simulink model "VCU_CS75_12_27_test"  (R2014a)
settings: Solver=FixedStepDiscrete  StartTime=0.0  StopTime=25  FixedStep=0.0005  RelTol=1e-3
undefined symbols (not defined in the file): D1, D2, D3, ecucoder_acal, ErrorSumMax1, ErrorSumMax2, ErrorSumMax3, I1, I2, I3, I_SW01_L, LaterlAngleCommand, LDW, P1, P2, P3, RemoteAcclPosition
libraries: simulink x913, ec5744lib x39
(part 26 of 30)

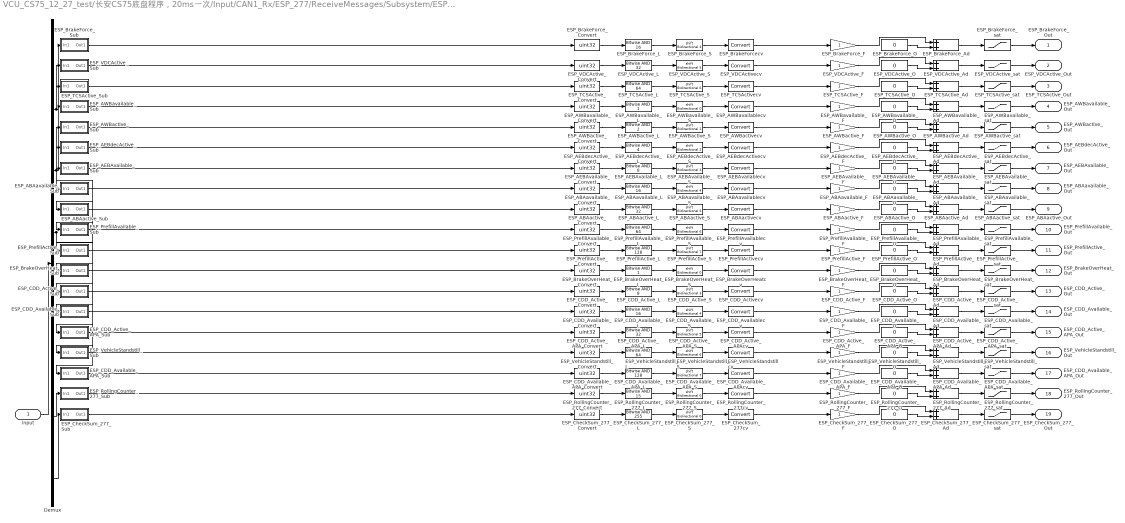
== system VCU_CS75_12_27_test/长安CS75底盘程序，20ms一次/Input/CAN1_Rx/ESP_277/ReceiveMessages/Subsystem/ESP_1 ==
  input : Inport
  Demux : Demux  Outputs=8
  ESP_ABAactive_Ad : Sum
  ESP_ABAactive_Convert : DataTypeConversion  OutDataTypeStr=uint32
  ESP_ABAactive_F : Gain
  ESP_ABAactive_L : simulink/Logic and Bit Operations/Bitwise Operator  logicop=AND  UseBitMask=on  BitMask=32  BitMaskRealWorld=Stored Integer
  ESP_ABAactive_O : Constant  Value=0  OutDataTypeStr=single
  ESP_ABAactive_S : ArithShift  BitShiftNumber=5
  ESP_ABAactive_Sub : Subsystem
  ESP_ABAactive_sat : Saturate  UpperLimit=1  LowerLimit=0
  ESP_ABAactivecv : DataTypeConversion
  ESP_ABAavailable_Ad : Sum
  ESP_ABAavailable_Convert : DataTypeConversion  OutDataTypeStr=uint32
  ESP_ABAavailable_F : Gain
  ESP_ABAavailable_L : simulink/Logic and Bit Operations/Bitwise Operator  logicop=AND  UseBitMask=on  BitMask=16  BitMaskRealWorld=Stored Integer
  ESP_ABAavailable_O : Constant  Value=0  OutDataTypeStr=single
  ESP_ABAavailable_S : ArithShift  BitShiftNumber=4
  ESP_ABAavailable_Sub : Subsystem
  ESP_ABAavailable_sat : Saturate  UpperLimit=1  LowerLimit=0
  ESP_ABAavailablecv : DataTypeConversion
  ESP_AEBAvailable_Ad : Sum
  ESP_AEBAvailable_Convert : DataTypeConversion  OutDataTypeStr=uint32
  ESP_AEBAvailable_F : Gain
  ESP_AEBAvailable_L : simulink/Logic and Bit Operations/Bitwise Operator  logicop=AND  UseBitMask=on  BitMask=8  BitMaskRealWorld=Stored Integer
  ESP_AEBAvailable_O : Constant  Value=0  OutDataTypeStr=single
  ESP_AEBAvailable_S : ArithShift  BitShiftNumber=3
  ESP_AEBAvailable_Sub : Subsystem
  ESP_AEBAvailable_sat : Saturate  UpperLimit=1  LowerLimit=0
  ESP_AEBAvailablecv : DataTypeConversion
  ESP_AEBdecActive_Ad : Sum
  ESP_AEBdecActive_Convert : DataTypeConversion  OutDataTypeStr=uint32
  ESP_AEBdecActive_F : Gain
  ESP_AEBdecActive_L : simulink/Logic and Bit Operations/Bitwise Operator  logicop=AND  UseBitMask=on  BitMask=4  BitMaskRealWorld=Stored Integer
  ESP_AEBdecActive_O : Constant  Value=0  OutDataTypeStr=single
  ESP_AEBdecActive_S : ArithShift  BitShiftNumber=2
  ESP_AEBdecActive_Sub : Subsystem
  ESP_AEBdecActive_sat : Saturate  UpperLimit=1  LowerLimit=0
  ESP_AEBdecActivecv : DataTypeConversion
  ESP_AWBactive_Ad : Sum
  ESP_AWBactive_Convert : DataTypeConversion  OutDataTypeStr=uint32
  ESP_AWBactive_F : Gain
  ESP_AWBactive_L : simulink/Logic and Bit Operations/Bitwise Operator  logicop=AND  UseBitMask=on  BitMask=2  BitMaskRealWorld=Stored Integer
  ESP_AWBactive_O : Constant  Value=0  OutDataTypeStr=single
  ESP_AWBactive_S : ArithShift  BitShiftNumber=1
  ESP_AWBactive_Sub : Subsystem
  ESP_AWBactive_sat : Saturate  UpperLimit=1  LowerLimit=0
  ESP_AWBactivecv : DataTypeConversion
  ESP_AWBavailable_Ad : Sum
  ESP_AWBavailable_Convert : DataTypeConversion  OutDataTypeStr=uint32
  ESP_AWBavailable_F : Gain
  ESP_AWBavailable_L : simulink/Logic and Bit Operations/Bitwise Operator  logicop=AND  UseBitMask=on  BitMask=1  BitMaskRealWorld=Stored Integer
  ESP_AWBavailable_O : Constant  Value=0  OutDataTypeStr=single
  ESP_AWBavailable_S : ArithShift
  ESP_AWBavailable_Sub : Subsystem
  ESP_AWBavailable_sat : Saturate  UpperLimit=1  LowerLimit=0
  ESP_AWBavailablecv : DataTypeConversion
  ESP_BrakeForce_Ad : Sum
  ESP_BrakeForce_Convert : DataTypeConversion  OutDataTypeStr=uint32
  ESP_BrakeForce_F : Gain
  ESP_BrakeForce_L : simulink/Logic and Bit Operations/Bitwise Operator  logicop=AND  UseBitMask=on  BitMask=16  BitMaskRealWorld=Stored Integer
  ESP_BrakeForce_O : Constant  Value=0  OutDataTypeStr=single
  ESP_BrakeForce_S : ArithShift  BitShiftNumber=4
  ESP_BrakeForce_Sub : Subsystem
  ESP_BrakeForce_sat : Saturate  UpperLimit=1  LowerLimit=0
  ESP_BrakeForcecv : DataTypeConversion
  ESP_BrakeOverHeat_Ad : Sum
  ESP_BrakeOverHeat_Convert : DataTypeConversion  OutDataTypeStr=uint32
  ESP_BrakeOverHeat_F : Gain
  ESP_BrakeOverHeat_L : simulink/Logic and Bit Operations/Bitwise Operator  logicop=AND  UseBitMask=on  BitMask=1  BitMaskRealWorld=Stored Integer
  ESP_BrakeOverHeat_O : Constant  Value=0  OutDataTypeStr=single
  ESP_BrakeOverHeat_S : ArithShift
  ESP_BrakeOverHeat_Sub : Subsystem
  ESP_BrakeOverHeat_sat : Saturate  UpperLimit=1  LowerLimit=0
  ESP_BrakeOverHeatcv : DataTypeConversion
  ESP_CDD_Active_APA_Ad : Sum
  ESP_CDD_Active_APA_Convert : DataTypeConversion  OutDataTypeStr=uint32
  ESP_CDD_Active_APA_F : Gain
  ESP_CDD_Active_APA_L : simulink/Logic and Bit Operations/Bitwise Operator  logicop=AND  UseBitMask=on  BitMask=32  BitMaskRealWorld=Stored Integer
  ESP_CDD_Active_APA_O : Constant  Value=0  OutDataTypeStr=single
  ESP_CDD_Active_APA_S : ArithShift  BitShiftNumber=5
  ESP_CDD_Active_APA_Sub : Subsystem
  ESP_CDD_Active_APA_sat : Saturate  UpperLimit=0  LowerLimit=0
  ESP_CDD_Active_APAcv : DataTypeConversion
  ESP_CDD_Active_Ad : Sum
  ESP_CDD_Active_Convert : DataTypeConversion  OutDataTypeStr=uint32
  ESP_CDD_Active_F : Gain
  ESP_CDD_Active_L : simulink/Logic and Bit Operations/Bitwise Operator  logicop=AND  UseBitMask=on  BitMask=8  BitMaskRealWorld=Stored Integer
  ESP_CDD_Active_O : Constant  Value=0  OutDataTypeStr=single
  ESP_CDD_Active_S : ArithShift  BitShiftNumber=3
  ESP_CDD_Active_Sub : Subsystem
  ESP_CDD_Active_sat : Saturate  UpperLimit=1  LowerLimit=0
  ESP_CDD_Activecv : DataTypeConversion
  ESP_CDD_Available_APA_Ad : Sum
  ESP_CDD_Available_APA_Convert : DataTypeConversion  OutDataTypeStr=uint32
  ESP_CDD_Available_APA_F : Gain
  ESP_CDD_Available_APA_L : simulink/Logic and Bit Operations/Bitwise Operator  logicop=AND  UseBitMask=on  BitMask=128  BitMaskRealWorld=Stored Integer
  ESP_CDD_Available_APA_O : Constant  Value=0  OutDataTypeStr=single
  ESP_CDD_Available_APA_S : ArithShift  BitShiftNumber=7
  ESP_CDD_Available_APA_Sub : Subsystem
  ESP_CDD_Available_APA_sat : Saturate  UpperLimit=0  LowerLimit=0
  ESP_CDD_Available_APAcv : DataTypeConversion
  ESP_CDD_Available_Ad : Sum
  ESP_CDD_Available_Convert : DataTypeConversion  OutDataTypeStr=uint32
  ESP_CDD_Available_F : Gain
  ESP_CDD_Available_L : simulink/Logic and Bit Operations/Bitwise Operator  logicop=AND  UseBitMask=on  BitMask=16  BitMaskRealWorld=Stored Integer
  ESP_CDD_Available_O : Constant  Value=0  OutDataTypeStr=single
  ESP_CDD_Available_S : ArithShift  BitShiftNumber=4
  ESP_CDD_Available_Sub : Subsystem
  ESP_CDD_Available_sat : Saturate  UpperLimit=1  LowerLimit=0
  ESP_CDD_Availablecv : DataTypeConversion
  ESP_CheckSum_277_Ad : Sum
  ESP_CheckSum_277_Convert : DataTypeConversion  OutDataTypeStr=uint32
  ESP_CheckSum_277_F : Gain
  ESP_CheckSum_277_L : simulink/Logic and Bit Operations/Bitwise Operator  logicop=AND  UseBitMask=on  BitMask=255  BitMaskRealWorld=Stored Integer
  ESP_CheckSum_277_O : Constant  Value=0  OutDataTypeStr=single
  ESP_CheckSum_277_S : ArithShift
  ESP_CheckSum_277_Sub : Subsystem
  ESP_CheckSum_277_sat : Saturate  UpperLimit=255  LowerLimit=0
  ESP_CheckSum_277cv : DataTypeConversion
  ESP_PrefillActive_Ad : Sum
  ESP_PrefillActive_Convert : DataTypeConversion  OutDataTypeStr=uint32
  ESP_PrefillActive_F : Gain
  ESP_PrefillActive_L : simulink/Logic and Bit Operations/Bitwise Operator  logicop=AND  UseBitMask=on  BitMask=128  BitMaskRealWorld=Stored Integer
  ESP_PrefillActive_O : Constant  Value=0  OutDataTypeStr=single
  ESP_PrefillActive_S : ArithShift  BitShiftNumber=7
  ESP_PrefillActive_Sub : Subsystem
  ESP_PrefillActive_sat : Saturate  UpperLimit=1  LowerLimit=0
  ESP_PrefillActivecv : DataTypeConversion
  ESP_PrefillAvailable_Ad : Sum
  ESP_PrefillAvailable_Convert : DataTypeConversion  OutDataTypeStr=uint32
  ESP_PrefillAvailable_F : Gain
  ESP_PrefillAvailable_L : simulink/Logic and Bit Operations/Bitwise Operator  logicop=AND  UseBitMask=on  BitMask=64  BitMaskRealWorld=Stored Integer
  ESP_PrefillAvailable_O : Constant  Value=0  OutDataTypeStr=single
  ESP_PrefillAvailable_S : ArithShift  BitShiftNumber=6
  ESP_PrefillAvailable_Sub : Subsystem
  ESP_PrefillAvailable_sat : Saturate  UpperLimit=1  LowerLimit=0
  ESP_PrefillAvailablecv : DataTypeConversion
  ESP_RollingCounter_277_Ad : Sum
  ESP_RollingCounter_277_Convert : DataTypeConversion  OutDataTypeStr=uint32
  ESP_RollingCounter_277_F : Gain
  ESP_RollingCounter_277_L : simulink/Logic and Bit Operations/Bitwise Operator  logicop=AND  UseBitMask=on  BitMask=15  BitMaskRealWorld=Stored Integer
  ESP_RollingCounter_277_O : Constant  Value=0  OutDataTypeStr=single
  ESP_RollingCounter_277_S : ArithShift
  ESP_RollingCounter_277_Sub : Subsystem
  ESP_RollingCounter_277_sat : Saturate  UpperLimit=15  LowerLimit=0
  ESP_RollingCounter_277cv : DataTypeConversion
  ESP_TCSActive_Ad : Sum
  ESP_TCSActive_Convert : DataTypeConversion  OutDataTypeStr=uint32
  ESP_TCSActive_F : Gain
  ESP_TCSActive_L : simulink/Logic and Bit Operations/Bitwise Operator  logicop=AND  UseBitMask=on  BitMask=64  BitMaskRealWorld=Stored Integer
  ESP_TCSActive_O : Constant  Value=0  OutDataTypeStr=single
  ESP_TCSActive_S : ArithShift  BitShiftNumber=6
  ESP_TCSActive_Sub : Subsystem
  ESP_TCSActive_sat : Saturate  UpperLimit=1  LowerLimit=0
  ESP_TCSActivecv : DataTypeConversion
  ESP_VDCActive_Ad : Sum
  ESP_VDCActive_Convert : DataTypeConversion  OutDataTypeStr=uint32
  ESP_VDCActive_F : Gain
  ESP_VDCActive_L : simulink/Logic and Bit Operations/Bitwise Operator  logicop=AND  UseBitMask=on  BitMask=32  BitMaskRealWorld=Stored Integer
  ESP_VDCActive_O : Constant  Value=0  OutDataTypeStr=single
  ESP_VDCActive_S : ArithShift  BitShiftNumber=5
  ESP_VDCActive_Sub : Subsystem
  ESP_VDCActive_sat : Saturate  UpperLimit=1  LowerLimit=0
  ESP_VDCActivecv : DataTypeConversion
  ESP_VehicleStandstill_Ad : Sum
  ESP_VehicleStandstill_Convert : DataTypeConversion  OutDataTypeStr=uint32
  ESP_VehicleStandstill_F : Gain
  ESP_VehicleStandstill_L : simulink/Logic and Bit Operations/Bitwise Operator  logicop=AND  UseBitMask=on  BitMask=64  BitMaskRealWorld=Stored Integer
  ESP_VehicleStandstill_O : Constant  Value=0  OutDataTypeStr=single
  ESP_VehicleStandstill_S : ArithShift  BitShiftNumber=6
  ESP_VehicleStandstill_Sub : Subsystem
  ESP_VehicleStandstill_sat : Saturate  UpperLimit=1  LowerLimit=0
  ESP_VehicleStandstillcv : DataTypeConversion
  ESP_BrakeForce_Out : Outport
  ESP_VDCActive_Out : Outport  Port=2
  ESP_TCSActive_Out : Outport  Port=3
  ESP_AWBavailable_Out : Outport  Port=4
  ESP_AWBactive_Out : Outport  Port=5
  ESP_AEBdecActive_Out : Outport  Port=6
  ESP_AEBAvailable_Out : Outport  Port=7
  ESP_ABAavailable_Out : Outport  Port=8
  ESP_ABAactive_Out : Outport  Port=9
  ESP_PrefillAvailable_Out : Outport  Port=10
  ESP_PrefillActive_Out : Outport  Port=11
  ESP_BrakeOverHeat_Out : Outport  Port=12
  ESP_CDD_Active_Out : Outport  Port=13
  ESP_CDD_Available_Out : Outport  Port=14
  ESP_CDD_Active_APA_Out : Outport  Port=15
  ESP_VehicleStandstill_Out : Outport  Port=16
  ESP_CDD_Available_APA_Out : Outport  Port=17
  ESP_RollingCounter_277_Out : Outport  Port=18
  ESP_CheckSum_277_Out : Outport  Port=19
  wires:
  input/1 -> Demux/1
  ESP_CheckSum_277cv/1 -> ESP_CheckSum_277_F/1
  ESP_CheckSum_277_S/1 -> ESP_CheckSum_277cv/1
  ESP_CheckSum_277_L/1 -> ESP_CheckSum_277_S/1
  ESP_CheckSum_277_Convert/1 -> ESP_CheckSum_277_L/1
  ESP_CheckSum_277_Sub/1(Out1) -> ESP_CheckSum_277_Convert/1
  Demux/8 -> ESP_CheckSum_277_Sub/1(In1)
  ESP_CheckSum_277_sat/1 -> ESP_CheckSum_277_Out/1
  ESP_CheckSum_277_Ad/1 -> ESP_CheckSum_277_sat/1
  ESP_CheckSum_277_O/1 -> ESP_CheckSum_277_Ad/2
  ESP_CheckSum_277_F/1 -> ESP_CheckSum_277_Ad/1
  ESP_RollingCounter_277cv/1 -> ESP_RollingCounter_277_F/1
  ESP_RollingCounter_277_S/1 -> ESP_RollingCounter_277cv/1
  ESP_RollingCounter_277_L/1 -> ESP_RollingCounter_277_S/1
  ESP_RollingCounter_277_Convert/1 -> ESP_RollingCounter_277_L/1
  ESP_RollingCounter_277_Sub/1(Out1) -> ESP_RollingCounter_277_Convert/1
  Demux/7 -> ESP_RollingCounter_277_Sub/1(In1)
  ESP_RollingCounter_277_sat/1 -> ESP_RollingCounter_277_Out/1
  ESP_RollingCounter_277_Ad/1 -> ESP_RollingCounter_277_sat/1
  ESP_RollingCounter_277_O/1 -> ESP_RollingCounter_277_Ad/2
  ESP_RollingCounter_277_F/1 -> ESP_RollingCounter_277_Ad/1
  ESP_CDD_Available_APAcv/1 -> ESP_CDD_Available_APA_F/1
  ESP_CDD_Available_APA_S/1 -> ESP_CDD_Available_APAcv/1
  ESP_CDD_Available_APA_L/1 -> ESP_CDD_Available_APA_S/1
  ESP_CDD_Available_APA_Convert/1 -> ESP_CDD_Available_APA_L/1
  ESP_CDD_Available_APA_Sub/1(Out1) -> ESP_CDD_Available_APA_Convert/1
  ESP_CDD_Available_APA_sat/1 -> ESP_CDD_Available_APA_Out/1
  ESP_CDD_Available_APA_Ad/1 -> ESP_CDD_Available_APA_sat/1
  ESP_CDD_Available_APA_O/1 -> ESP_CDD_Available_APA_Ad/2
  ESP_CDD_Available_APA_F/1 -> ESP_CDD_Available_APA_Ad/1
  ESP_VehicleStandstillcv/1 -> ESP_VehicleStandstill_F/1
  ESP_VehicleStandstill_S/1 -> ESP_VehicleStandstillcv/1
  ESP_VehicleStandstill_L/1 -> ESP_VehicleStandstill_S/1
  ESP_VehicleStandstill_Convert/1 -> ESP_VehicleStandstill_L/1
  ESP_VehicleStandstill_Sub/1(Out1) -> ESP_VehicleStandstill_Convert/1
  ESP_VehicleStandstill_sat/1 -> ESP_VehicleStandstill_Out/1
  ESP_VehicleStandstill_Ad/1 -> ESP_VehicleStandstill_sat/1
  ESP_VehicleStandstill_O/1 -> ESP_VehicleStandstill_Ad/2
  ESP_VehicleStandstill_F/1 -> ESP_VehicleStandstill_Ad/1
  ESP_CDD_Active_APAcv/1 -> ESP_CDD_Active_APA_F/1
  ESP_CDD_Active_APA_S/1 -> ESP_CDD_Active_APAcv/1
  ESP_CDD_Active_APA_L/1 -> ESP_CDD_Active_APA_S/1
  ESP_CDD_Active_APA_Convert/1 -> ESP_CDD_Active_APA_L/1
  ESP_CDD_Active_APA_Sub/1(Out1) -> ESP_CDD_Active_APA_Convert/1
  ESP_CDD_Active_APA_sat/1 -> ESP_CDD_Active_APA_Out/1
  ESP_CDD_Active_APA_Ad/1 -> ESP_CDD_Active_APA_sat/1
  ESP_CDD_Active_APA_O/1 -> ESP_CDD_Active_APA_Ad/2
  ESP_CDD_Active_APA_F/1 -> ESP_CDD_Active_APA_Ad/1
  ESP_CDD_Availablecv/1 -> ESP_CDD_Available_F/1
  ESP_CDD_Available_S/1 -> ESP_CDD_Availablecv/1
  ESP_CDD_Available_L/1 -> ESP_CDD_Available_S/1
  ESP_CDD_Available_Convert/1 -> ESP_CDD_Available_L/1
  ESP_CDD_Available_Sub/1(Out1) -> ESP_CDD_Available_Convert/1
  ESP_CDD_Available_sat/1 -> ESP_CDD_Available_Out/1
  ESP_CDD_Available_Ad/1 -> ESP_CDD_Available_sat/1
  ESP_CDD_Available_O/1 -> ESP_CDD_Available_Ad/2
  ESP_CDD_Available_F/1 -> ESP_CDD_Available_Ad/1
  ESP_CDD_Activecv/1 -> ESP_CDD_Active_F/1
  ESP_CDD_Active_S/1 -> ESP_CDD_Activecv/1
  ESP_CDD_Active_L/1 -> ESP_CDD_Active_S/1
  ESP_CDD_Active_Convert/1 -> ESP_CDD_Active_L/1
  ESP_CDD_Active_Sub/1(Out1) -> ESP_CDD_Active_Convert/1
  ESP_CDD_Active_sat/1 -> ESP_CDD_Active_Out/1
  ESP_CDD_Active_Ad/1 -> ESP_CDD_Active_sat/1
  ESP_CDD_Active_O/1 -> ESP_CDD_Active_Ad/2
  ESP_CDD_Active_F/1 -> ESP_CDD_Active_Ad/1
  ESP_BrakeOverHeatcv/1 -> ESP_BrakeOverHeat_F/1
  ESP_BrakeOverHeat_S/1 -> ESP_BrakeOverHeatcv/1
  ESP_BrakeOverHeat_L/1 -> ESP_BrakeOverHeat_S/1
  ESP_BrakeOverHeat_Convert/1 -> ESP_BrakeOverHeat_L/1
  ESP_BrakeOverHeat_Sub/1(Out1) -> ESP_BrakeOverHeat_Convert/1
  Demux/4 -> ESP_CDD_Available_APA_Sub/1(In1), ESP_VehicleStandstill_Sub/1(In1), ESP_CDD_Active_APA_Sub/1(In1), ESP_CDD_Available_Sub/1(In1), ESP_CDD_Active_Sub/1(In1), ESP_BrakeOverHeat_Sub/1(In1)
  ESP_BrakeOverHeat_sat/1 -> ESP_BrakeOverHeat_Out/1
  ESP_BrakeOverHeat_Ad/1 -> ESP_BrakeOverHeat_sat/1
  ESP_BrakeOverHeat_O/1 -> ESP_BrakeOverHeat_Ad/2
  ESP_BrakeOverHeat_F/1 -> ESP_BrakeOverHeat_Ad/1
  ESP_PrefillActivecv/1 -> ESP_PrefillActive_F/1
  ESP_PrefillActive_S/1 -> ESP_PrefillActivecv/1
  ESP_PrefillActive_L/1 -> ESP_PrefillActive_S/1
  ESP_PrefillActive_Convert/1 -> ESP_PrefillActive_L/1
  ESP_PrefillActive_Sub/1(Out1) -> ESP_PrefillActive_Convert/1
  ESP_PrefillActive_sat/1 -> ESP_PrefillActive_Out/1
  ESP_PrefillActive_Ad/1 -> ESP_PrefillActive_sat/1
  ESP_PrefillActive_O/1 -> ESP_PrefillActive_Ad/2
  ESP_PrefillActive_F/1 -> ESP_PrefillActive_Ad/1
  ESP_PrefillAvailablecv/1 -> ESP_PrefillAvailable_F/1
  ESP_PrefillAvailable_S/1 -> ESP_PrefillAvailablecv/1
  ESP_PrefillAvailable_L/1 -> ESP_PrefillAvailable_S/1
  ESP_PrefillAvailable_Convert/1 -> ESP_PrefillAvailable_L/1
  ESP_PrefillAvailable_Sub/1(Out1) -> ESP_PrefillAvailable_Convert/1
  ESP_PrefillAvailable_sat/1 -> ESP_PrefillAvailable_Out/1
  ESP_PrefillAvailable_Ad/1 -> ESP_PrefillAvailable_sat/1
  ESP_PrefillAvailable_O/1 -> ESP_PrefillAvailable_Ad/2
  ESP_PrefillAvailable_F/1 -> ESP_PrefillAvailable_Ad/1
  ESP_ABAactivecv/1 -> ESP_ABAactive_F/1
  ESP_ABAactive_S/1 -> ESP_ABAactivecv/1
  ESP_ABAactive_L/1 -> ESP_ABAactive_S/1
  ESP_ABAactive_Convert/1 -> ESP_ABAactive_L/1
  ESP_ABAactive_Sub/1(Out1) -> ESP_ABAactive_Convert/1
  ESP_ABAactive_sat/1 -> ESP_ABAactive_Out/1
  ESP_ABAactive_Ad/1 -> ESP_ABAactive_sat/1
  ESP_ABAactive_O/1 -> ESP_ABAactive_Ad/2
  ESP_ABAactive_F/1 -> ESP_ABAactive_Ad/1
  ESP_ABAavailablecv/1 -> ESP_ABAavailable_F/1
  ESP_ABAavailable_S/1 -> ESP_ABAavailablecv/1
  ESP_ABAavailable_L/1 -> ESP_ABAavailable_S/1
  ESP_ABAavailable_Convert/1 -> ESP_ABAavailable_L/1
  ESP_ABAavailable_Sub/1(Out1) -> ESP_ABAavailable_Convert/1
  ESP_ABAavailable_sat/1 -> ESP_ABAavailable_Out/1
  ESP_ABAavailable_Ad/1 -> ESP_ABAavailable_sat/1
  ESP_ABAavailable_O/1 -> ESP_ABAavailable_Ad/2
  ESP_ABAavailable_F/1 -> ESP_ABAavailable_Ad/1
  ESP_AEBAvailablecv/1 -> ESP_AEBAvailable_F/1
  ESP_AEBAvailable_S/1 -> ESP_AEBAvailablecv/1
  ESP_AEBAvailable_L/1 -> ESP_AEBAvailable_S/1
  ESP_AEBAvailable_Convert/1 -> ESP_AEBAvailable_L/1
  ESP_AEBAvailable_Sub/1(Out1) -> ESP_AEBAvailable_Convert/1
  ESP_AEBAvailable_sat/1 -> ESP_AEBAvailable_Out/1
  ESP_AEBAvailable_Ad/1 -> ESP_AEBAvailable_sat/1
  ESP_AEBAvailable_O/1 -> ESP_AEBAvailable_Ad/2
  ESP_AEBAvailable_F/1 -> ESP_AEBAvailable_Ad/1
  ESP_AEBdecActivecv/1 -> ESP_AEBdecActive_F/1
  ESP_AEBdecActive_S/1 -> ESP_AEBdecActivecv/1
  ESP_AEBdecActive_L/1 -> ESP_AEBdecActive_S/1
  ESP_AEBdecActive_Convert/1 -> ESP_AEBdecActive_L/1
  ESP_AEBdecActive_Sub/1(Out1) -> ESP_AEBdecActive_Convert/1
  ESP_AEBdecActive_sat/1 -> ESP_AEBdecActive_Out/1
  ESP_AEBdecActive_Ad/1 -> ESP_AEBdecActive_sat/1
  ESP_AEBdecActive_O/1 -> ESP_AEBdecActive_Ad/2
  ESP_AEBdecActive_F/1 -> ESP_AEBdecActive_Ad/1
  ESP_AWBactivecv/1 -> ESP_AWBactive_F/1
  ESP_AWBactive_S/1 -> ESP_AWBactivecv/1
  ESP_AWBactive_L/1 -> ESP_AWBactive_S/1
  ESP_AWBactive_Convert/1 -> ESP_AWBactive_L/1
  ESP_AWBactive_Sub/1(Out1) -> ESP_AWBactive_Convert/1
  ESP_AWBactive_sat/1 -> ESP_AWBactive_Out/1
  ESP_AWBactive_Ad/1 -> ESP_AWBactive_sat/1
  ESP_AWBactive_O/1 -> ESP_AWBactive_Ad/2
  ESP_AWBactive_F/1 -> ESP_AWBactive_Ad/1
  ESP_AWBavailablecv/1 -> ESP_AWBavailable_F/1
  ESP_AWBavailable_S/1 -> ESP_AWBavailablecv/1
  ESP_AWBavailable_L/1 -> ESP_AWBavailable_S/1
  ESP_AWBavailable_Convert/1 -> ESP_AWBavailable_L/1
  ESP_AWBavailable_Sub/1(Out1) -> ESP_AWBavailable_Convert/1
  Demux/3 -> ESP_PrefillActive_Sub/1(In1), ESP_PrefillAvailable_Sub/1(In1), ESP_ABAactive_Sub/1(In1), ESP_ABAavailable_Sub/1(In1), ESP_AEBAvailable_Sub/1(In1), ESP_AEBdecActive_Sub/1(In1), ESP_AWBactive_Sub/1(In1), ESP_AWBavailable_Sub/1(In1)
  ESP_AWBavailable_sat/1 -> ESP_AWBavailable_Out/1
  ESP_AWBavailable_Ad/1 -> ESP_AWBavailable_sat/1
  ESP_AWBavailable_O/1 -> ESP_AWBavailable_Ad/2
  ESP_AWBavailable_F/1 -> ESP_AWBavailable_Ad/1
  ESP_TCSActivecv/1 -> ESP_TCSActive_F/1
  ESP_TCSActive_S/1 -> ESP_TCSActivecv/1
  ESP_TCSActive_L/1 -> ESP_TCSActive_S/1
  ESP_TCSActive_Convert/1 -> ESP_TCSActive_L/1
  ESP_TCSActive_Sub/1(Out1) -> ESP_TCSActive_Convert/1
  ESP_TCSActive_sat/1 -> ESP_TCSActive_Out/1
  ESP_TCSActive_Ad/1 -> ESP_TCSActive_sat/1
  ESP_TCSActive_O/1 -> ESP_TCSActive_Ad/2
  ESP_TCSActive_F/1 -> ESP_TCSActive_Ad/1
  ESP_VDCActivecv/1 -> ESP_VDCActive_F/1
  ESP_VDCActive_S/1 -> ESP_VDCActivecv/1
  ESP_VDCActive_L/1 -> ESP_VDCActive_S/1
  ESP_VDCActive_Convert/1 -> ESP_VDCActive_L/1
  ESP_VDCActive_Sub/1(Out1) -> ESP_VDCActive_Convert/1
  ESP_VDCActive_sat/1 -> ESP_VDCActive_Out/1
  ESP_VDCActive_Ad/1 -> ESP_VDCActive_sat/1
  ESP_VDCActive_O/1 -> ESP_VDCActive_Ad/2
  ESP_VDCActive_F/1 -> ESP_VDCActive_Ad/1
  ESP_BrakeForcecv/1 -> ESP_BrakeForce_F/1
  ESP_BrakeForce_S/1 -> ESP_BrakeForcecv/1
  ESP_BrakeForce_L/1 -> ESP_BrakeForce_S/1
  ESP_BrakeForce_Convert/1 -> ESP_BrakeForce_L/1
  ESP_BrakeForce_Sub/1(Out1) -> ESP_BrakeForce_Convert/1
  Demux/2 -> ESP_TCSActive_Sub/1(In1), ESP_VDCActive_Sub/1(In1), ESP_BrakeForce_Sub/1(In1)
  ESP_BrakeForce_sat/1 -> ESP_BrakeForce_Out/1
  ESP_BrakeForce_Ad/1 -> ESP_BrakeForce_sat/1
  ESP_BrakeForce_O/1 -> ESP_BrakeForce_Ad/2
  ESP_BrakeForce_F/1 -> ESP_BrakeForce_Ad/1

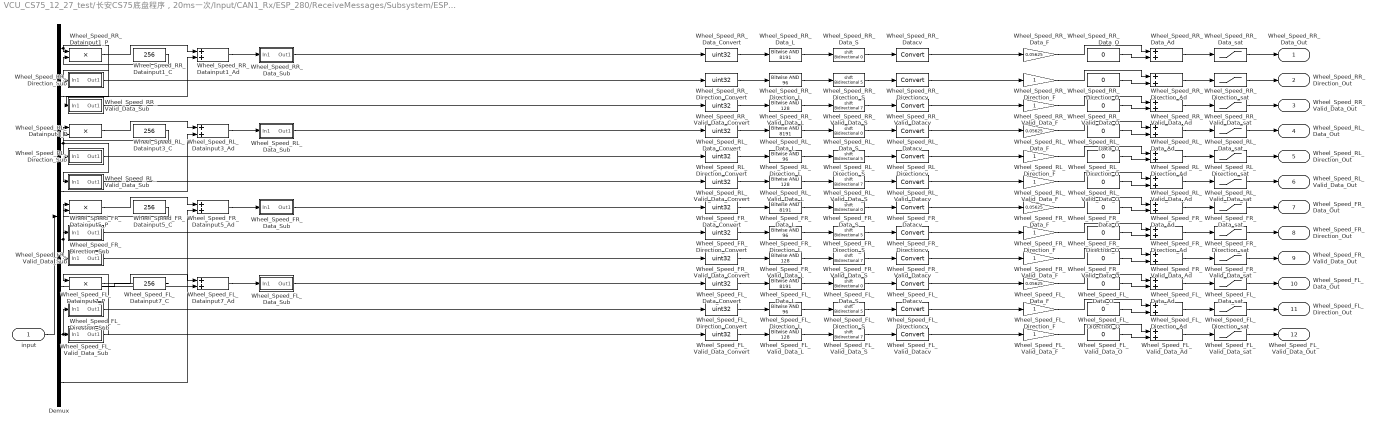
== system VCU_CS75_12_27_test/长安CS75底盘程序，20ms一次/Input/CAN1_Rx/ESP_280/ReceiveMessages/Subsystem/ESP_1 ==
  input : Inport
  Demux : Demux  Outputs=8
  Wheel_Speed_FL_Data_Ad : Sum
  Wheel_Speed_FL_Data_Convert : DataTypeConversion  OutDataTypeStr=uint32
  Wheel_Speed_FL_Data_F : Gain  Gain=0.05625
  Wheel_Speed_FL_Data_L : simulink/Logic and Bit Operations/Bitwise Operator  logicop=AND  UseBitMask=on  BitMask=8191  BitMaskRealWorld=Stored Integer
  Wheel_Speed_FL_Data_O : Constant  Value=0  OutDataTypeStr=single
  Wheel_Speed_FL_Data_S : ArithShift
  Wheel_Speed_FL_Data_Sub : Subsystem
  Wheel_Speed_FL_Data_sat : Saturate  UpperLimit=360  LowerLimit=0
  Wheel_Speed_FL_Datacv : DataTypeConversion
  Wheel_Speed_FL_Datainput7_Ad : Sum
  Wheel_Speed_FL_Datainput7_C : Constant  Value=256
  Wheel_Speed_FL_Datainput7_P : Product
  Wheel_Speed_FL_Direction_Ad : Sum
  Wheel_Speed_FL_Direction_Convert : DataTypeConversion  OutDataTypeStr=uint32
  Wheel_Speed_FL_Direction_F : Gain
  Wheel_Speed_FL_Direction_L : simulink/Logic and Bit Operations/Bitwise Operator  logicop=AND  UseBitMask=on  BitMask=96  BitMaskRealWorld=Stored Integer
  Wheel_Speed_FL_Direction_O : Constant  Value=0  OutDataTypeStr=single
  Wheel_Speed_FL_Direction_S : ArithShift  BitShiftNumber=5
  Wheel_Speed_FL_Direction_Sub : Subsystem
  Wheel_Speed_FL_Direction_sat : Saturate  UpperLimit=3  LowerLimit=0
  Wheel_Speed_FL_Directioncv : DataTypeConversion
  Wheel_Speed_FL_Valid_Data_Ad : Sum
  Wheel_Speed_FL_Valid_Data_Convert : DataTypeConversion  OutDataTypeStr=uint32
  Wheel_Speed_FL_Valid_Data_F : Gain
  Wheel_Speed_FL_Valid_Data_L : simulink/Logic and Bit Operations/Bitwise Operator  logicop=AND  UseBitMask=on  BitMask=128  BitMaskRealWorld=Stored Integer
  Wheel_Speed_FL_Valid_Data_O : Constant  Value=0  OutDataTypeStr=single
  Wheel_Speed_FL_Valid_Data_S : ArithShift  BitShiftNumber=7
  Wheel_Speed_FL_Valid_Data_Sub : Subsystem
  Wheel_Speed_FL_Valid_Data_sat : Saturate  UpperLimit=1  LowerLimit=0
  Wheel_Speed_FL_Valid_Datacv : DataTypeConversion
  Wheel_Speed_FR_Data_Ad : Sum
  Wheel_Speed_FR_Data_Convert : DataTypeConversion  OutDataTypeStr=uint32
  Wheel_Speed_FR_Data_F : Gain  Gain=0.05625
  Wheel_Speed_FR_Data_L : simulink/Logic and Bit Operations/Bitwise Operator  logicop=AND  UseBitMask=on  BitMask=8191  BitMaskRealWorld=Stored Integer
  Wheel_Speed_FR_Data_O : Constant  Value=0  OutDataTypeStr=single
  Wheel_Speed_FR_Data_S : ArithShift
  Wheel_Speed_FR_Data_Sub : Subsystem
  Wheel_Speed_FR_Data_sat : Saturate  UpperLimit=360  LowerLimit=0
  Wheel_Speed_FR_Datacv : DataTypeConversion
  Wheel_Speed_FR_Datainput5_Ad : Sum
  Wheel_Speed_FR_Datainput5_C : Constant  Value=256
  Wheel_Speed_FR_Datainput5_P : Product
  Wheel_Speed_FR_Direction_Ad : Sum
  Wheel_Speed_FR_Direction_Convert : DataTypeConversion  OutDataTypeStr=uint32
  Wheel_Speed_FR_Direction_F : Gain
  Wheel_Speed_FR_Direction_L : simulink/Logic and Bit Operations/Bitwise Operator  logicop=AND  UseBitMask=on  BitMask=96  BitMaskRealWorld=Stored Integer
  Wheel_Speed_FR_Direction_O : Constant  Value=0  OutDataTypeStr=single
  Wheel_Speed_FR_Direction_S : ArithShift  BitShiftNumber=5
  Wheel_Speed_FR_Direction_Sub : Subsystem
  Wheel_Speed_FR_Direction_sat : Saturate  UpperLimit=3  LowerLimit=0
  Wheel_Speed_FR_Directioncv : DataTypeConversion
  Wheel_Speed_FR_Valid_Data_Ad : Sum
  Wheel_Speed_FR_Valid_Data_Convert : DataTypeConversion  OutDataTypeStr=uint32
  Wheel_Speed_FR_Valid_Data_F : Gain
  Wheel_Speed_FR_Valid_Data_L : simulink/Logic and Bit Operations/Bitwise Operator  logicop=AND  UseBitMask=on  BitMask=128  BitMaskRealWorld=Stored Integer
  Wheel_Speed_FR_Valid_Data_O : Constant  Value=0  OutDataTypeStr=single
  Wheel_Speed_FR_Valid_Data_S : ArithShift  BitShiftNumber=7
  Wheel_Speed_FR_Valid_Data_Sub : Subsystem
  Wheel_Speed_FR_Valid_Data_sat : Saturate  UpperLimit=1  LowerLimit=0
  Wheel_Speed_FR_Valid_Datacv : DataTypeConversion
  Wheel_Speed_RL_Data_Ad : Sum
  Wheel_Speed_RL_Data_Convert : DataTypeConversion  OutDataTypeStr=uint32
  Wheel_Speed_RL_Data_F : Gain  Gain=0.05625
  Wheel_Speed_RL_Data_L : simulink/Logic and Bit Operations/Bitwise Operator  logicop=AND  UseBitMask=on  BitMask=8191  BitMaskRealWorld=Stored Integer
  Wheel_Speed_RL_Data_O : Constant  Value=0  OutDataTypeStr=single
  Wheel_Speed_RL_Data_S : ArithShift
  Wheel_Speed_RL_Data_Sub : Subsystem
  Wheel_Speed_RL_Data_sat : Saturate  UpperLimit=360  LowerLimit=0
  Wheel_Speed_RL_Datacv : DataTypeConversion
  Wheel_Speed_RL_Datainput3_Ad : Sum
  Wheel_Speed_RL_Datainput3_C : Constant  Value=256
  Wheel_Speed_RL_Datainput3_P : Product
  Wheel_Speed_RL_Direction_Ad : Sum
  Wheel_Speed_RL_Direction_Convert : DataTypeConversion  OutDataTypeStr=uint32
  Wheel_Speed_RL_Direction_F : Gain
  Wheel_Speed_RL_Direction_L : simulink/Logic and Bit Operations/Bitwise Operator  logicop=AND  UseBitMask=on  BitMask=96  BitMaskRealWorld=Stored Integer
  Wheel_Speed_RL_Direction_O : Constant  Value=0  OutDataTypeStr=single
  Wheel_Speed_RL_Direction_S : ArithShift  BitShiftNumber=5
  Wheel_Speed_RL_Direction_Sub : Subsystem
  Wheel_Speed_RL_Direction_sat : Saturate  UpperLimit=3  LowerLimit=0
  Wheel_Speed_RL_Directioncv : DataTypeConversion
  Wheel_Speed_RL_Valid_Data_Ad : Sum
  Wheel_Speed_RL_Valid_Data_Convert : DataTypeConversion  OutDataTypeStr=uint32
  Wheel_Speed_RL_Valid_Data_F : Gain
  Wheel_Speed_RL_Valid_Data_L : simulink/Logic and Bit Operations/Bitwise Operator  logicop=AND  UseBitMask=on  BitMask=128  BitMaskRealWorld=Stored Integer
  Wheel_Speed_RL_Valid_Data_O : Constant  Value=0  OutDataTypeStr=single
  Wheel_Speed_RL_Valid_Data_S : ArithShift  BitShiftNumber=7
  Wheel_Speed_RL_Valid_Data_Sub : Subsystem
  Wheel_Speed_RL_Valid_Data_sat : Saturate  UpperLimit=1  LowerLimit=0
  Wheel_Speed_RL_Valid_Datacv : DataTypeConversion
  Wheel_Speed_RR_Data_Ad : Sum
  Wheel_Speed_RR_Data_Convert : DataTypeConversion  OutDataTypeStr=uint32
  Wheel_Speed_RR_Data_F : Gain  Gain=0.05625
  Wheel_Speed_RR_Data_L : simulink/Logic and Bit Operations/Bitwise Operator  logicop=AND  UseBitMask=on  BitMask=8191  BitMaskRealWorld=Stored Integer
  Wheel_Speed_RR_Data_O : Constant  Value=0  OutDataTypeStr=single
  Wheel_Speed_RR_Data_S : ArithShift
  Wheel_Speed_RR_Data_Sub : Subsystem
  Wheel_Speed_RR_Data_sat : Saturate  UpperLimit=360  LowerLimit=0
  Wheel_Speed_RR_Datacv : DataTypeConversion
  Wheel_Speed_RR_Datainput1_Ad : Sum
  Wheel_Speed_RR_Datainput1_C : Constant  Value=256
  Wheel_Speed_RR_Datainput1_P : Product
  Wheel_Speed_RR_Direction_Ad : Sum
  Wheel_Speed_RR_Direction_Convert : DataTypeConversion  OutDataTypeStr=uint32
  Wheel_Speed_RR_Direction_F : Gain
  Wheel_Speed_RR_Direction_L : simulink/Logic and Bit Operations/Bitwise Operator  logicop=AND  UseBitMask=on  BitMask=96  BitMaskRealWorld=Stored Integer
  Wheel_Speed_RR_Direction_O : Constant  Value=0  OutDataTypeStr=single
  Wheel_Speed_RR_Direction_S : ArithShift  BitShiftNumber=5
  Wheel_Speed_RR_Direction_Sub : Subsystem
  Wheel_Speed_RR_Direction_sat : Saturate  UpperLimit=3  LowerLimit=0
  Wheel_Speed_RR_Directioncv : DataTypeConversion
  Wheel_Speed_RR_Valid_Data_Ad : Sum
  Wheel_Speed_RR_Valid_Data_Convert : DataTypeConversion  OutDataTypeStr=uint32
  Wheel_Speed_RR_Valid_Data_F : Gain
  Wheel_Speed_RR_Valid_Data_L : simulink/Logic and Bit Operations/Bitwise Operator  logicop=AND  UseBitMask=on  BitMask=128  BitMaskRealWorld=Stored Integer
  Wheel_Speed_RR_Valid_Data_O : Constant  Value=0  OutDataTypeStr=single
  Wheel_Speed_RR_Valid_Data_S : ArithShift  BitShiftNumber=7
  Wheel_Speed_RR_Valid_Data_Sub : Subsystem
  Wheel_Speed_RR_Valid_Data_sat : Saturate  UpperLimit=1  LowerLimit=0
  Wheel_Speed_RR_Valid_Datacv : DataTypeConversion
  Wheel_Speed_RR_Data_Out : Outport
  Wheel_Speed_RR_Direction_Out : Outport  Port=2
  Wheel_Speed_RR_Valid_Data_Out : Outport  Port=3
  Wheel_Speed_RL_Data_Out : Outport  Port=4
  Wheel_Speed_RL_Direction_Out : Outport  Port=5
  Wheel_Speed_RL_Valid_Data_Out : Outport  Port=6
  Wheel_Speed_FR_Data_Out : Outport  Port=7
  Wheel_Speed_FR_Direction_Out : Outport  Port=8
  Wheel_Speed_FR_Valid_Data_Out : Outport  Port=9
  Wheel_Speed_FL_Data_Out : Outport  Port=10
  Wheel_Speed_FL_Direction_Out : Outport  Port=11
  Wheel_Speed_FL_Valid_Data_Out : Outport  Port=12
  wires:
  input/1 -> Demux/1
  Wheel_Speed_FL_Valid_Datacv/1 -> Wheel_Speed_FL_Valid_Data_F/1
  Wheel_Speed_FL_Valid_Data_S/1 -> Wheel_Speed_FL_Valid_Datacv/1
  Wheel_Speed_FL_Valid_Data_L/1 -> Wheel_Speed_FL_Valid_Data_S/1
  Wheel_Speed_FL_Valid_Data_Convert/1 -> Wheel_Speed_FL_Valid_Data_L/1
  Wheel_Speed_FL_Valid_Data_Sub/1(Out1) -> Wheel_Speed_FL_Valid_Data_Convert/1
  Wheel_Speed_FL_Valid_Data_sat/1 -> Wheel_Speed_FL_Valid_Data_Out/1
  Wheel_Speed_FL_Valid_Data_Ad/1 -> Wheel_Speed_FL_Valid_Data_sat/1
  Wheel_Speed_FL_Valid_Data_O/1 -> Wheel_Speed_FL_Valid_Data_Ad/2
  Wheel_Speed_FL_Valid_Data_F/1 -> Wheel_Speed_FL_Valid_Data_Ad/1
  Wheel_Speed_FL_Directioncv/1 -> Wheel_Speed_FL_Direction_F/1
  Wheel_Speed_FL_Direction_S/1 -> Wheel_Speed_FL_Directioncv/1
  Wheel_Speed_FL_Direction_L/1 -> Wheel_Speed_FL_Direction_S/1
  Wheel_Speed_FL_Direction_Convert/1 -> Wheel_Speed_FL_Direction_L/1
  Wheel_Speed_FL_Direction_Sub/1(Out1) -> Wheel_Speed_FL_Direction_Convert/1
  Wheel_Speed_FL_Direction_sat/1 -> Wheel_Speed_FL_Direction_Out/1
  Wheel_Speed_FL_Direction_Ad/1 -> Wheel_Speed_FL_Direction_sat/1
  Wheel_Speed_FL_Direction_O/1 -> Wheel_Speed_FL_Direction_Ad/2
  Wheel_Speed_FL_Direction_F/1 -> Wheel_Speed_FL_Direction_Ad/1
  Wheel_Speed_FL_Datacv/1 -> Wheel_Speed_FL_Data_F/1
  Wheel_Speed_FL_Data_S/1 -> Wheel_Speed_FL_Datacv/1
  Wheel_Speed_FL_Data_L/1 -> Wheel_Speed_FL_Data_S/1
  Wheel_Speed_FL_Data_Convert/1 -> Wheel_Speed_FL_Data_L/1
  Wheel_Speed_FL_Data_Sub/1(Out1) -> Wheel_Speed_FL_Data_Convert/1
  Wheel_Speed_FL_Datainput7_Ad/1 -> Wheel_Speed_FL_Data_Sub/1(In1)
  Demux/8 -> Wheel_Speed_FL_Datainput7_Ad/2
  Wheel_Speed_FL_Datainput7_P/1 -> Wheel_Speed_FL_Datainput7_Ad/1
  Wheel_Speed_FL_Datainput7_C/1 -> Wheel_Speed_FL_Datainput7_P/2
  Demux/7 -> Wheel_Speed_FL_Valid_Data_Sub/1(In1), Wheel_Speed_FL_Direction_Sub/1(In1), Wheel_Speed_FL_Datainput7_P/1
  Wheel_Speed_FL_Data_sat/1 -> Wheel_Speed_FL_Data_Out/1
  Wheel_Speed_FL_Data_Ad/1 -> Wheel_Speed_FL_Data_sat/1
  Wheel_Speed_FL_Data_O/1 -> Wheel_Speed_FL_Data_Ad/2
  Wheel_Speed_FL_Data_F/1 -> Wheel_Speed_FL_Data_Ad/1
  Wheel_Speed_FR_Valid_Datacv/1 -> Wheel_Speed_FR_Valid_Data_F/1
  Wheel_Speed_FR_Valid_Data_S/1 -> Wheel_Speed_FR_Valid_Datacv/1
  Wheel_Speed_FR_Valid_Data_L/1 -> Wheel_Speed_FR_Valid_Data_S/1
  Wheel_Speed_FR_Valid_Data_Convert/1 -> Wheel_Speed_FR_Valid_Data_L/1
  Wheel_Speed_FR_Valid_Data_Sub/1(Out1) -> Wheel_Speed_FR_Valid_Data_Convert/1
  Wheel_Speed_FR_Valid_Data_sat/1 -> Wheel_Speed_FR_Valid_Data_Out/1
  Wheel_Speed_FR_Valid_Data_Ad/1 -> Wheel_Speed_FR_Valid_Data_sat/1
  Wheel_Speed_FR_Valid_Data_O/1 -> Wheel_Speed_FR_Valid_Data_Ad/2
  Wheel_Speed_FR_Valid_Data_F/1 -> Wheel_Speed_FR_Valid_Data_Ad/1
  Wheel_Speed_FR_Directioncv/1 -> Wheel_Speed_FR_Direction_F/1
  Wheel_Speed_FR_Direction_S/1 -> Wheel_Speed_FR_Directioncv/1
  Wheel_Speed_FR_Direction_L/1 -> Wheel_Speed_FR_Direction_S/1
  Wheel_Speed_FR_Direction_Convert/1 -> Wheel_Speed_FR_Direction_L/1
  Wheel_Speed_FR_Direction_Sub/1(Out1) -> Wheel_Speed_FR_Direction_Convert/1
  Wheel_Speed_FR_Direction_sat/1 -> Wheel_Speed_FR_Direction_Out/1
  Wheel_Speed_FR_Direction_Ad/1 -> Wheel_Speed_FR_Direction_sat/1
  Wheel_Speed_FR_Direction_O/1 -> Wheel_Speed_FR_Direction_Ad/2
  Wheel_Speed_FR_Direction_F/1 -> Wheel_Speed_FR_Direction_Ad/1
  Wheel_Speed_FR_Datacv/1 -> Wheel_Speed_FR_Data_F/1
  Wheel_Speed_FR_Data_S/1 -> Wheel_Speed_FR_Datacv/1
  Wheel_Speed_FR_Data_L/1 -> Wheel_Speed_FR_Data_S/1
  Wheel_Speed_FR_Data_Convert/1 -> Wheel_Speed_FR_Data_L/1
  Wheel_Speed_FR_Data_Sub/1(Out1) -> Wheel_Speed_FR_Data_Convert/1
  Wheel_Speed_FR_Datainput5_Ad/1 -> Wheel_Speed_FR_Data_Sub/1(In1)
  Demux/6 -> Wheel_Speed_FR_Datainput5_Ad/2
  Wheel_Speed_FR_Datainput5_P/1 -> Wheel_Speed_FR_Datainput5_Ad/1
  Wheel_Speed_FR_Datainput5_C/1 -> Wheel_Speed_FR_Datainput5_P/2
  Demux/5 -> Wheel_Speed_FR_Valid_Data_Sub/1(In1), Wheel_Speed_FR_Direction_Sub/1(In1), Wheel_Speed_FR_Datainput5_P/1
  Wheel_Speed_FR_Data_sat/1 -> Wheel_Speed_FR_Data_Out/1
  Wheel_Speed_FR_Data_Ad/1 -> Wheel_Speed_FR_Data_sat/1
  Wheel_Speed_FR_Data_O/1 -> Wheel_Speed_FR_Data_Ad/2
  Wheel_Speed_FR_Data_F/1 -> Wheel_Speed_FR_Data_Ad/1
  Wheel_Speed_RL_Valid_Datacv/1 -> Wheel_Speed_RL_Valid_Data_F/1
  Wheel_Speed_RL_Valid_Data_S/1 -> Wheel_Speed_RL_Valid_Datacv/1
  Wheel_Speed_RL_Valid_Data_L/1 -> Wheel_Speed_RL_Valid_Data_S/1
  Wheel_Speed_RL_Valid_Data_Convert/1 -> Wheel_Speed_RL_Valid_Data_L/1
  Wheel_Speed_RL_Valid_Data_Sub/1(Out1) -> Wheel_Speed_RL_Valid_Data_Convert/1
  Wheel_Speed_RL_Valid_Data_sat/1 -> Wheel_Speed_RL_Valid_Data_Out/1
  Wheel_Speed_RL_Valid_Data_Ad/1 -> Wheel_Speed_RL_Valid_Data_sat/1
  Wheel_Speed_RL_Valid_Data_O/1 -> Wheel_Speed_RL_Valid_Data_Ad/2
  Wheel_Speed_RL_Valid_Data_F/1 -> Wheel_Speed_RL_Valid_Data_Ad/1
  Wheel_Speed_RL_Directioncv/1 -> Wheel_Speed_RL_Direction_F/1
  Wheel_Speed_RL_Direction_S/1 -> Wheel_Speed_RL_Directioncv/1
  Wheel_Speed_RL_Direction_L/1 -> Wheel_Speed_RL_Direction_S/1
  Wheel_Speed_RL_Direction_Convert/1 -> Wheel_Speed_RL_Direction_L/1
  Wheel_Speed_RL_Direction_Sub/1(Out1) -> Wheel_Speed_RL_Direction_Convert/1
  Wheel_Speed_RL_Direction_sat/1 -> Wheel_Speed_RL_Direction_Out/1
  Wheel_Speed_RL_Direction_Ad/1 -> Wheel_Speed_RL_Direction_sat/1
  Wheel_Speed_RL_Direction_O/1 -> Wheel_Speed_RL_Direction_Ad/2
  Wheel_Speed_RL_Direction_F/1 -> Wheel_Speed_RL_Direction_Ad/1
  Wheel_Speed_RL_Datacv/1 -> Wheel_Speed_RL_Data_F/1
  Wheel_Speed_RL_Data_S/1 -> Wheel_Speed_RL_Datacv/1
  Wheel_Speed_RL_Data_L/1 -> Wheel_Speed_RL_Data_S/1
  Wheel_Speed_RL_Data_Convert/1 -> Wheel_Speed_RL_Data_L/1
  Wheel_Speed_RL_Data_Sub/1(Out1) -> Wheel_Speed_RL_Data_Convert/1
  Wheel_Speed_RL_Datainput3_Ad/1 -> Wheel_Speed_RL_Data_Sub/1(In1)
  Demux/4 -> Wheel_Speed_RL_Datainput3_Ad/2
  Wheel_Speed_RL_Datainput3_P/1 -> Wheel_Speed_RL_Datainput3_Ad/1
  Wheel_Speed_RL_Datainput3_C/1 -> Wheel_Speed_RL_Datainput3_P/2
  Demux/3 -> Wheel_Speed_RL_Valid_Data_Sub/1(In1), Wheel_Speed_RL_Direction_Sub/1(In1), Wheel_Speed_RL_Datainput3_P/1
  Wheel_Speed_RL_Data_sat/1 -> Wheel_Speed_RL_Data_Out/1
  Wheel_Speed_RL_Data_Ad/1 -> Wheel_Speed_RL_Data_sat/1
  Wheel_Speed_RL_Data_O/1 -> Wheel_Speed_RL_Data_Ad/2
  Wheel_Speed_RL_Data_F/1 -> Wheel_Speed_RL_Data_Ad/1
  Wheel_Speed_RR_Valid_Datacv/1 -> Wheel_Speed_RR_Valid_Data_F/1
  Wheel_Speed_RR_Valid_Data_S/1 -> Wheel_Speed_RR_Valid_Datacv/1
  Wheel_Speed_RR_Valid_Data_L/1 -> Wheel_Speed_RR_Valid_Data_S/1
  Wheel_Speed_RR_Valid_Data_Convert/1 -> Wheel_Speed_RR_Valid_Data_L/1
  Wheel_Speed_RR_Valid_Data_Sub/1(Out1) -> Wheel_Speed_RR_Valid_Data_Convert/1
  Wheel_Speed_RR_Valid_Data_sat/1 -> Wheel_Speed_RR_Valid_Data_Out/1
  Wheel_Speed_RR_Valid_Data_Ad/1 -> Wheel_Speed_RR_Valid_Data_sat/1
  Wheel_Speed_RR_Valid_Data_O/1 -> Wheel_Speed_RR_Valid_Data_Ad/2
  Wheel_Speed_RR_Valid_Data_F/1 -> Wheel_Speed_RR_Valid_Data_Ad/1
  Wheel_Speed_RR_Directioncv/1 -> Wheel_Speed_RR_Direction_F/1
  Wheel_Speed_RR_Direction_S/1 -> Wheel_Speed_RR_Directioncv/1
  Wheel_Speed_RR_Direction_L/1 -> Wheel_Speed_RR_Direction_S/1
  Wheel_Speed_RR_Direction_Convert/1 -> Wheel_Speed_RR_Direction_L/1
  Wheel_Speed_RR_Direction_Sub/1(Out1) -> Wheel_Speed_RR_Direction_Convert/1
  Wheel_Speed_RR_Direction_sat/1 -> Wheel_Speed_RR_Direction_Out/1
  Wheel_Speed_RR_Direction_Ad/1 -> Wheel_Speed_RR_Direction_sat/1
  Wheel_Speed_RR_Direction_O/1 -> Wheel_Speed_RR_Direction_Ad/2
  Wheel_Speed_RR_Direction_F/1 -> Wheel_Speed_RR_Direction_Ad/1
  Wheel_Speed_RR_Datacv/1 -> Wheel_Speed_RR_Data_F/1
  Wheel_Speed_RR_Data_S/1 -> Wheel_Speed_RR_Datacv/1
  Wheel_Speed_RR_Data_L/1 -> Wheel_Speed_RR_Data_S/1
  Wheel_Speed_RR_Data_Convert/1 -> Wheel_Speed_RR_Data_L/1
  Wheel_Speed_RR_Data_Sub/1(Out1) -> Wheel_Speed_RR_Data_Convert/1
  Wheel_Speed_RR_Datainput1_Ad/1 -> Wheel_Speed_RR_Data_Sub/1(In1)
  Demux/2 -> Wheel_Speed_RR_Datainput1_Ad/2
  Wheel_Speed_RR_Datainput1_P/1 -> Wheel_Speed_RR_Datainput1_Ad/1
  Wheel_Speed_RR_Datainput1_C/1 -> Wheel_Speed_RR_Datainput1_P/2
  Demux/1 -> Wheel_Speed_RR_Valid_Data_Sub/1(In1), Wheel_Speed_RR_Direction_Sub/1(In1), Wheel_Speed_RR_Datainput1_P/1
  Wheel_Speed_RR_Data_sat/1 -> Wheel_Speed_RR_Data_Out/1
  Wheel_Speed_RR_Data_Ad/1 -> Wheel_Speed_RR_Data_sat/1
  Wheel_Speed_RR_Data_O/1 -> Wheel_Speed_RR_Data_Ad/2
  Wheel_Speed_RR_Data_F/1 -> Wheel_Speed_RR_Data_Ad/1
